simulink model "PPC_P2"  (R2019b)
settings: Solver=VariableStepAuto  StartTime=0.0  StopTime=50.0  RelTol=1e-3
undefined symbols (not defined in the file): sigbuilder_block
libraries: slctrlblks x2, simulink x1
settings Model: Creator=Kevin  LastModifiedBy=Kevin

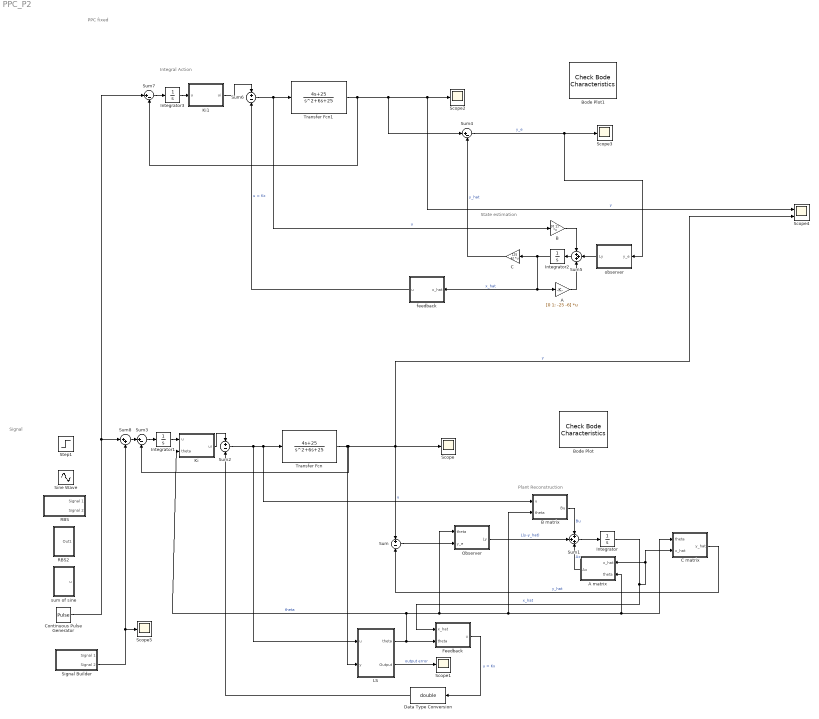
== system PPC_P2 ==
  note: PPC fixed
  note: Plant Reconstruction
  note: Signal
  note: Integral Action
  note: State estimation
  A : Gain  Gain=[0 1; -25 -6]  Multiplication=Matrix(K*u)
  A matrix : MATLAB Function  TreatAsAtomicUnit=on
  B : Gain  Gain=[0 1]'  Multiplication=Matrix(K*u)
  B matrix : MATLAB Function  TreatAsAtomicUnit=on
  Bode Plot : slctrlblks/Model Verification/Check Bode  Characteristics  InstantiateOnLoad=on  SaveOperatingPoints=off  LinearizationIOs={'/Sum2', 1, 'in', 'on', '';'/Transfer Fcn', 1, 'out', 'on', ''}  LinearizeAt=SnapshotTimes  SnapshotTimes=[0]  TriggerType=rising  SampleTime=auto  RateConversionMethod=zoh  PreWarpFreq=10  UseExactDelayModel=off  UseFullBlockNameLabels=off  UseBusSignalLabels=off  enabled=on  stopWhenAssertionFail=off  export=off  ViewDlgPos=[1921 -319 1920 967.333333333333]  OpenViewOnLoad=off  LaunchViewOnOpen=off  FrequencyUnits=rad/s  MagnitudeUnits=dB  PhaseUnits=deg  TimeUnits=seconds  EnableUpperBound=off  UpperBoundFrequencies=[]  UpperBoundMagnitudes=[]  EnableLowerBound=off  LowerBoundFrequencies=[]  LowerBoundMagnitudes=[]
      settings: SourceProductName=Simulink Control Design
  Bode Plot1 : slctrlblks/Model Verification/Check Bode  Characteristics  InstantiateOnLoad=on  SaveOperatingPoints=off  LinearizationIOs={'/Sum2', 1, 'in', 'off', '';'/Transfer Fcn', 1, 'out', 'on', ''}  LinearizeAt=SnapshotTimes  SnapshotTimes=[0]  TriggerType=rising  SampleTime=auto  RateConversionMethod=zoh  PreWarpFreq=10  UseExactDelayModel=off  UseFullBlockNameLabels=off  UseBusSignalLabels=off  enabled=on  stopWhenAssertionFail=off  export=off  ViewDlgPos=[1921 -319 1920 967.333333333333]  OpenViewOnLoad=off  LaunchViewOnOpen=off  FrequencyUnits=rad/s  MagnitudeUnits=dB  PhaseUnits=deg  TimeUnits=seconds  EnableUpperBound=off  UpperBoundFrequencies=[]  UpperBoundMagnitudes=[]  EnableLowerBound=off  LowerBoundFrequencies=[]  LowerBoundMagnitudes=[]
      settings: SourceProductName=Simulink Control Design
  C : Gain  Gain=[25 4]  Multiplication=Matrix(K*u)
  C matrix : MATLAB Function  TreatAsAtomicUnit=on
  Continuous Pulse Generator : DiscretePulseGenerator  PulseType=Time based  Period=1  PulseWidth=50
  Data Type Conversion : DataTypeConversion  OutDataTypeStr=double
  Feedback : MATLAB Function  TreatAsAtomicUnit=on
  Integrator{,1..3} (4 alike) : Integrator
  Ki : MATLAB Function  TreatAsAtomicUnit=on
  Ki1 : MATLAB Function  TreatAsAtomicUnit=on
  LS : Subsystem
  "Observer " : MATLAB Function  TreatAsAtomicUnit=on
  "RBS " : Subsystem  Tag=STV Subsys  LoadFcn=sigbuilder_block('load');  StartFcn=sigbuilder_block('start');  StopFcn=sigbuilder_block('stop');  ClipboardFcn=sigbuilder_block('clipboard');  mask(Sigbuilder block){tuvar=[0:10]}
      mask help: Simulink:masks:SigbuilderBlock_MD
      mask init:
      | if ~strcmp(get_param(bdroot(gcbh),'SimulationStatus'),'stopped') tuvar = sigbuilder_block('maskInit'); end
      settings: CopyFcn=sigbuilder_block('copy');  DeleteFcn=sigbuilder_block('delete');  ModelCloseFcn=sigbuilder_block('modelClose');  PreSaveFcn=sigbuilder_block('preSave');  PauseFcn=sigbuilder_block('pause');  ContinueFcn=sigbuilder_block('continue');  NameChangeFcn=sigbuilder_block('namechange');  OpenFcn=sigbuilder_block('open',[215 62.5 550.5 362.5 ]);  CloseFcn=sigbuilder_block('close');
      mask Display: plot(0, 0, 100, 100,[2, 2, 32, 32, 2], [68, 8, 8, 68, 68],[32, 2], [38, 38], [32, 19, 2],[53, 60, 44], [32, 17, 17, 2],[16, 16, 31, 31]);txt = getActiveGroup(gcbh);text(2, 100, txt,'verticalAlignment', 'top');
  RBS2 : Subsystem
  Scope{,1..3,5} (5 alike) : Scope
  Scope4 : Scope  NumInputPorts=2
  Signal Builder : Subsystem  Tag=STV Subsys  LoadFcn=sigbuilder_block('load',[242.5 79.5 550.5 362.5 ]);  StartFcn=sigbuilder_block('start');  StopFcn=sigbuilder_block('stop');  ClipboardFcn=sigbuilder_block('clipboard');  mask(Sigbuilder block){tuvar=[0:10]}
      mask help: Simulink:masks:SigbuilderBlock_MD
      mask init:
      | if ~strcmp(get_param(bdroot(gcbh),'SimulationStatus'),'stopped') tuvar = sigbuilder_block('maskInit'); end
      settings: CopyFcn=sigbuilder_block('copy');  DeleteFcn=sigbuilder_block('delete');  ModelCloseFcn=sigbuilder_block('modelClose');  PreSaveFcn=sigbuilder_block('preSave');  PauseFcn=sigbuilder_block('pause');  ContinueFcn=sigbuilder_block('continue');  NameChangeFcn=sigbuilder_block('namechange');  OpenFcn=sigbuilder_block('open',[216 79 550.5 362.5 ]);  CloseFcn=sigbuilder_block('close');
      mask Display: plot(0, 0, 100, 100,[2, 2, 32, 32, 2], [68, 8, 8, 68, 68],[32, 2], [38, 38], [32, 19, 2],[53, 60, 44], [32, 17, 17, 2],[16, 16, 31, 31]);txt = getActiveGroup(gcbh);text(2, 100, txt,'verticalAlignment', 'top');
  Sine Wave : Sin  Frequency=0.1  SampleTime=0
  Step1 : Step  SampleTime=0
  Sum : Sum  Inputs=+-
  Sum1 : Sum  Inputs=+++
  Sum2 : Sum  Inputs=+-
  Sum3 : Sum  Inputs=|+-
  Sum4 : Sum  Inputs=|+-
  Sum5 : Sum  Inputs=+++
  Sum6 : Sum  Inputs=+-
  Sum7 : Sum  Inputs=|+-
  Sum8 : Sum  Inputs=|++
  Transfer Fcn : TransferFcn  Numerator=[4 25]  Denominator=[1 ,6 ,25]
  Transfer Fcn1 : TransferFcn  Numerator=[4 25]  Denominator=[1 ,6 ,25]
  feedback : MATLAB Function  TreatAsAtomicUnit=on
  "observer " : MATLAB Function  TreatAsAtomicUnit=on
  sum of sine : Subsystem
  wires:
  "Observer "/1(Ly) -> Sum1/2  "L(y-y_hat)"
  LS/2(Output) -> Scope1/1  "output error"
  B matrix/1(Bu) -> Sum1/1  "Bu"
  Sum1/1 -> Integrator/1
  LS/1(theta) -> C matrix/1(theta), A matrix/2(theta), B matrix/2(theta), "Observer "/1(theta), Ki/2(theta), Feedback/2(theta)  "theta"
  A matrix/1(Ax) -> Sum1/3  "Ax"
  Integrator/1 -> C matrix/2(x_hat), A matrix/1(x_hat), Feedback/1(x_hat)  "x_hat"
  Sum2/1 -> LS/1("u "), B matrix/1(u), Transfer Fcn/1  "u"
  Sum/1 -> "Observer "/2(y_e)
  Transfer Fcn/1 -> Sum/1, Scope4/2, Scope/1, Sum3/2, LS/2(y)  "y"
  Feedback/1(u) -> Data Type Conversion/1  "u = Kx"
  C matrix/1(y_hat) -> Sum/2  "y_hat"
  Data Type Conversion/1 -> Sum2/2
  Sum3/1 -> Integrator1/1
  Integrator1/1 -> Ki/1(u)
  Ki/1(ui) -> Sum2/1
  feedback/1(u) -> Sum6/2  "u = Kx"
  Sum4/1 -> "observer "/1(y_e), Scope3/1  "y_e"
  Ki1/1(ui) -> Sum6/1
  Integrator3/1 -> Ki1/1(u)
  Transfer Fcn1/1 -> Sum4/1, Scope4/1, Scope2/1, Sum7/2  "y"
  A/1 -> Sum5/3
  Integrator2/1 -> C/1, feedback/1(x_hat), A/1  "x_hat"
  Sum5/1 -> Integrator2/1
  C/1 -> Sum4/2  "y_hat"
  "observer "/1(Ly) -> Sum5/2
  Sum7/1 -> Integrator3/1
  B/1 -> Sum5/1
  Continuous Pulse Generator/1 -> Sum8/1, Sum7/1
  Sum6/1 -> B/1, Transfer Fcn1/1  "u"
  Sum8/1 -> Sum3/1
  Signal Builder/2(Signal 2) -> Scope5/1, Sum8/2

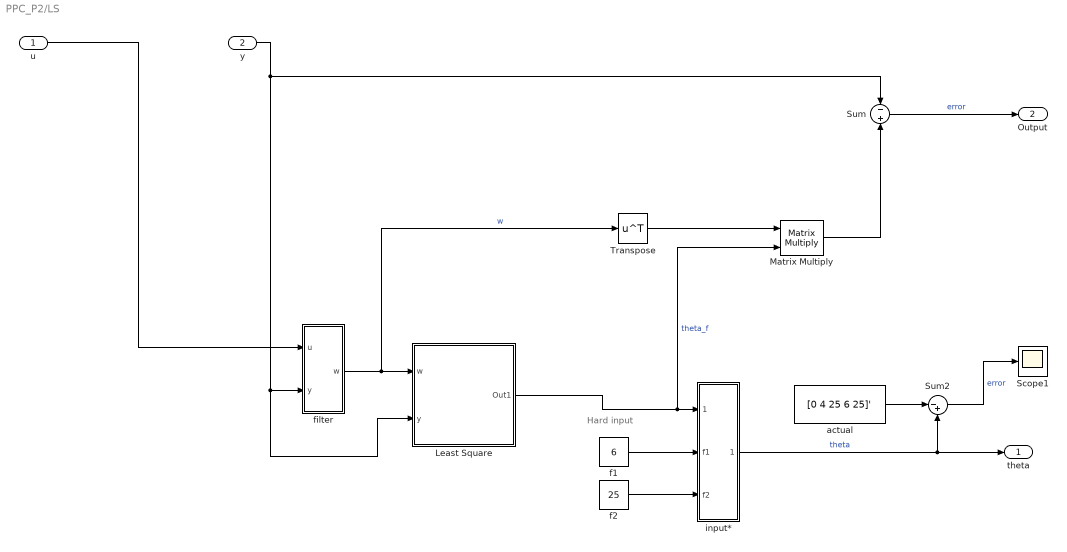
== system PPC_P2/LS ==
  note: Hard input
  "u " : Inport
  y : Inport  Port=2
  Least Square : Subsystem
  Matrix Multiply : Product  Multiplication=Matrix(*)
  Scope1 : Scope
  Sum : Sum  Inputs=-+
  Sum2 : Sum  Inputs=|-+
  Transpose : Math  Operator=transpose  SignedPower=off  SaturateOnIntegerOverflow=on
  actual : Constant  Value=[0 4 25 6 25]'
  f1 : Constant  Value=6
  f2 : Constant  Value=25
  "filter " : Subsystem
  input* : Subsystem
  theta : Outport
  Output : Outport  Port=2
  wires:
  y/1 -> Sum/1, Least Square/2(y), "filter "/2("y ")
  Sum2/1 -> Scope1/1  "error"
  f2/1 -> input*/3(f2)
  actual/1 -> Sum2/1
  "u "/1 -> "filter "/1("u ")
  f1/1 -> input*/2(f1)
  Least Square/1(Out1) -> Matrix Multiply/2, input*/1(theta_f)  "theta_f"
  input*/1(Out1) -> Sum2/2, theta/1  "theta"
  "filter "/1(w) -> Transpose/1, Least Square/1(w)  "w"
  Transpose/1 -> Matrix Multiply/1
  Matrix Multiply/1 -> Sum/2
  Sum/1 -> Output/1  "error"

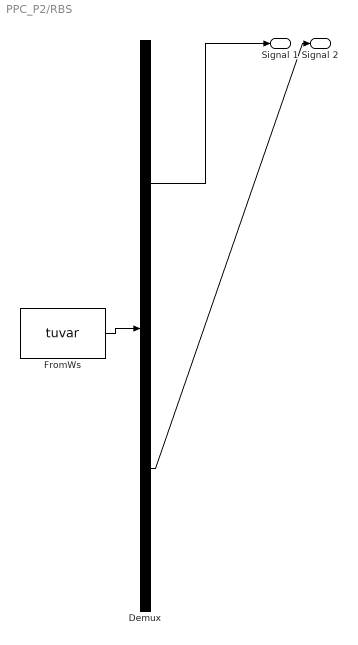
== system PPC_P2/RBS  ==
  Demux : Demux  Tag=STV Demux  Outputs=2
  FromWs : FromWorkspace  Tag=STV FromWs  VariableName=tuvar  SampleTime=0
      SigBuilderData=|
      | common.afterFinalStr = 'Extrapolate'
      | common.sampleTime = 0
      | dataSet.timeRange = [0 10]
      | dataSet.name = 'Group 1'
      | sbobj.Groups.Name = 'Group 1'
      | sbobj.Groups.Signals(1).Name = 'Signal 1'
      | sbobj.Groups.Signals(1).XData = [0 4 4 6 6 10]
      | sbobj.Groups.Signals(1).YData = [0 0 1 1 0 0]
      | sbobj.Groups.Signals(2).Name = 'Signal 2'
      | sbobj.Groups.Signals(2).XData = [0 0.2 0.2 0.3 0.3 0.5 0.5 0.7 0.7 1 1 1.1 1.1 1.3 1.3 1.4 1.4 1.5 1.5 1.7 1.7 2.1 2.1 2.2 2.2 2.7 2.7 2.8 2.8 2.9 2.9 3 3 3.1 3.1 3.5 3.5 3.7 3.7 3.8 3.8 3.9 3.9 4.2 4.2 4.4 4.4 4.7 4.7 5 5 5.1 5.1 5.3 5.3 5.6 5.6 5.7 5.7 5.8 5.8 5.9 5.9 6 6 6.1 6.1 6.2 6.2 6.7 6.7 7 7 7.1 7.1 7.2 7.2 7.3 7.3 7.4 7.4 7.5 7.5 7.8 7.8 7.9 7.9 8.1 8.1 8.5 8.5 8.6 8.6 8.8 8.8 8.9 8.9 9 9 9.2 9.2 9.5 9.5 9.6 9.6 9.7 9.7 10]
      | sbobj.Groups.Signals(2).YData = [1 1 0 0 1 1 0 0 1 1 0 0 1 1 0 0 1 1 0 0 1 1 0 0 1 1 0 0 1 1 0 0 1 1 0 0 1 1 0 0 1 1 0 0 1 1 0 0 1 1 0 0 1 1 0 0 1 1 0 0 1 1 0 0 1 1 0 0 1 1 0 0 1 1 0 0 1 1 0 0 1 1 0 0 1 1 0 0 1 1 0 0 1 1 0 0 1 1 0 0 1 1 0 0 1 1 0 0]
  Signal 1 : Outport  Tag=STV Outport
  Signal 2 : Outport  Tag=STV Outport  Port=2
  wires:
  Demux/1 -> Signal 1/1
  FromWs/1 -> Demux/1
  Demux/2 -> Signal 2/1

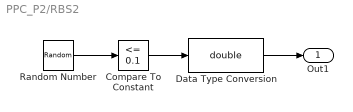
== system PPC_P2/RBS2 ==
  Compare To Constant : simulink/Logic and Bit Operations/Compare To Constant  relop=<=  const=0.1  OutDataTypeStr=boolean
  Data Type Conversion : DataTypeConversion  OutDataTypeStr=double
  Random Number : RandomNumber  Mean=1  SampleTime=10
  Out1 : Outport
  wires:
  Random Number/1 -> Compare To Constant/1
  Compare To Constant/1 -> Data Type Conversion/1
  Data Type Conversion/1 -> Out1/1

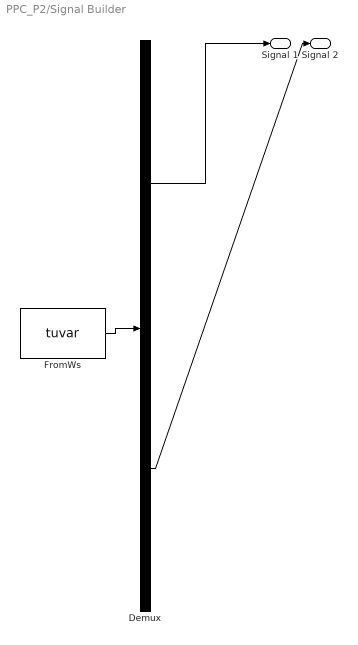
== system PPC_P2/Signal Builder ==
  Demux : Demux  Tag=STV Demux  Outputs=2
  FromWs : FromWorkspace  Tag=STV FromWs  VariableName=tuvar  SampleTime=0
      SigBuilderData=|
      | common.afterFinalStr = 'Extrapolate'
      | common.sampleTime = 0
      | dataSet.timeRange = [0 10]
      | dataSet.name = 'Group 1'
      | sbobj.Groups.Name = 'Group 1'
      | sbobj.Groups.Signals(1).Name = 'Signal 1'
      | sbobj.Groups.Signals(1).XData = [0 4 4 6 6 10]
      | sbobj.Groups.Signals(1).YData = [0 0 1 1 0 0]
      | sbobj.Groups.Signals(2).Name = 'Signal 2'
      | sbobj.Groups.Signals(2).XData = [0 0.25 0.5 0.75 1 1.25 1.5 1.75 2 2.25 2.5 2.75 3 3.25 3.5 3.75 4 4.25 4.5 4.75 5 5.25 5.5 5.75 6 6.25 6.5 6.75 7 7.25 7.5 7.75 8 8.25 8.5 8.75 9 9.25 9.5 9.75 10]
      | sbobj.Groups.Signals(2).YData = [0.0121419340162 -0.0764190690584 -0.164320775559 0.502978184919 0.351900863104 -0.0567183942106 0.0259717929394 0.453768030385 0.537981216054 0.330786163264 -0.0977542366685 -0.174844476245 0.225476170998 -0.259120295299 -0.321262673984 -0.106571039605 0.286763871566 0.0477844956174 0.0734825422898 0.33742490315 0.0703883754895 -0.341568743769 0.252628091547 0.142902550846 -0.0265169068696 -0.123910688666 -0.16337499212 -0.00720200578647 -0.240154097162 -0.153657109632 -0.446002612072 -0.155592567203 -0.207968715344 0.173295533063 0.436490088667 0.310645454952 0.314047045754 0.202863163156 0.16397838294 0.224996602257 -0.218951692736]
  Signal 1 : Outport  Tag=STV Outport
  Signal 2 : Outport  Tag=STV Outport  Port=2
  wires:
  Demux/1 -> Signal 1/1
  FromWs/1 -> Demux/1
  Demux/2 -> Signal 2/1

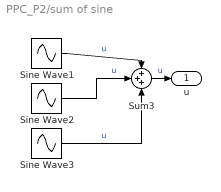
== system PPC_P2/sum of sine ==
  Sine Wave1 : Sin  Frequency=0.1  Phase=0.1  SampleTime=0
  Sine Wave2 : Sin  SampleTime=0
  Sine Wave3 : Sin  Frequency=2  SampleTime=0
  Sum3 : Sum  Inputs=+++
  u : Outport
  wires:
  Sine Wave3/1 -> Sum3/3  "u"
  Sine Wave1/1 -> Sum3/1  "u"
  Sum3/1 -> u/1  "u"
  Sine Wave2/1 -> Sum3/2  "u"

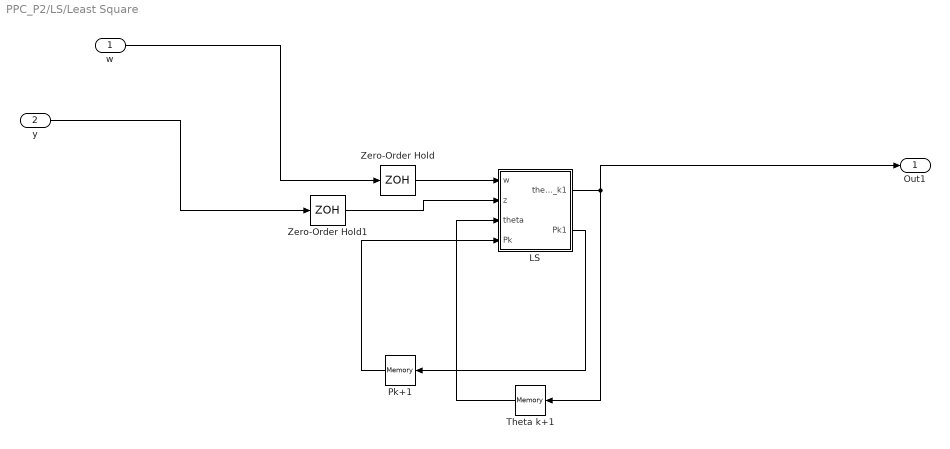
== system PPC_P2/LS/Least Square ==
  w : Inport
  y : Inport  Port=2
  LS : MATLAB Function  TreatAsAtomicUnit=on
  Pk+1 : Memory  InitialCondition=(10^5)*eye(5)  InheritSampleTime=on
  Theta k+1 : Memory  InitialCondition=[0 4.4 27.5 0.1 0.1]'  InheritSampleTime=on
  Zero-Order Hold : ZeroOrderHold  SampleTime=0.01
  Zero-Order Hold1 : ZeroOrderHold  SampleTime=0.01
  Out1 : Outport
  wires:
  Zero-Order Hold/1 -> LS/1(w)
  Pk+1/1 -> LS/4(Pk)
  Zero-Order Hold1/1 -> LS/2(z)
  LS/1(theta_k1) -> Out1/1, Theta k+1/1
  y/1 -> Zero-Order Hold1/1
  LS/2(Pk1) -> Pk+1/1
  Theta k+1/1 -> LS/3(theta)
  w/1 -> Zero-Order Hold/1

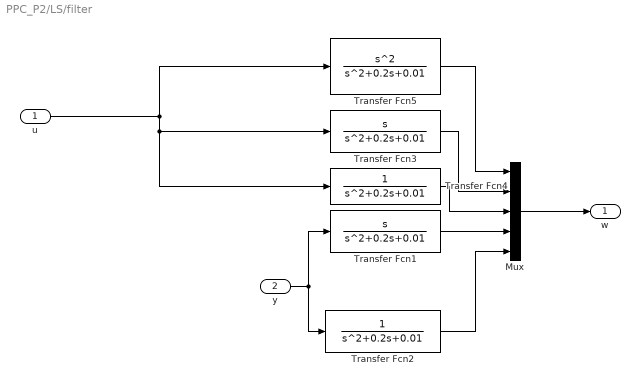
== system PPC_P2/LS/filter  ==
  "u " : Inport
  "y " : Inport  Port=2
  Mux : Mux  Inputs=5
  Transfer Fcn1 : TransferFcn  Numerator=[1 0]  Denominator=[1 0.2 0.01]
  Transfer Fcn2 : TransferFcn  Denominator=[1 0.2 0.01]
  Transfer Fcn3 : TransferFcn  Numerator=[1 0]  Denominator=[1 0.2 0.01]
  Transfer Fcn4 : TransferFcn  Denominator=[1 0.2 0.01]
  Transfer Fcn5 : TransferFcn  Numerator=[1 0 0]  Denominator=[1 0.2 0.01]
  w : Outport
  wires:
  Transfer Fcn1/1 -> Mux/4
  "u "/1 -> Transfer Fcn4/1, Transfer Fcn3/1, Transfer Fcn5/1
  Mux/1 -> w/1
  "y "/1 -> Transfer Fcn1/1, Transfer Fcn2/1
  Transfer Fcn2/1 -> Mux/5
  Transfer Fcn5/1 -> Mux/1
  Transfer Fcn3/1 -> Mux/2
  Transfer Fcn4/1 -> Mux/3

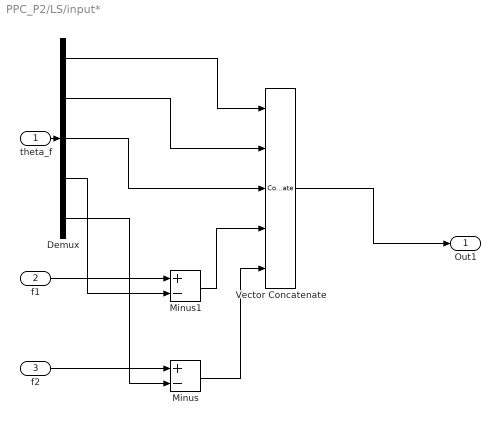
== system PPC_P2/LS/input* ==
  theta_f : Inport
  f1 : Inport  Port=2
  f2 : Inport  Port=3
  Demux : Demux  Outputs=5
  Minus : Sum  Inputs=+-
  Minus1 : Sum  Inputs=+-
  Vector Concatenate : Concatenate  NumInputs=5
  Out1 : Outport
  wires:
  Vector Concatenate/1 -> Out1/1
  Minus1/1 -> Vector Concatenate/4
  Minus/1 -> Vector Concatenate/5
  Demux/1 -> Vector Concatenate/1
  Demux/4 -> Minus1/2
  Demux/3 -> Vector Concatenate/3
  Demux/5 -> Minus/2
  f2/1 -> Minus/1
  Demux/2 -> Vector Concatenate/2
  f1/1 -> Minus1/1
  theta_f/1 -> Demux/1

== matlab function PPC_P2/LS/Least Square/LS ==
  data: w input; z input; theta input; Pk input; theta_k1 output; Pk1 output
function [ theta_k1,Pk1] = fcn(w, z, theta, Pk)
alpha = 1.4; %standard
gamma = 1/alpha;
%e = 10^-4;
%Q = e*eye(5);
%Pk = eye(5);

%initial values
%ro = 10^5;
%P1 = ro*eye(5);
%theta1 = [0 0 1 0.2 0.01]';
%Calculations

theta_k1 = theta - (gamma*Pk*w*(w'*theta-z))/ (1+gamma*w'*Pk*w);
Pk1 = (1/alpha)*Pk - ((gamma^2*Pk*w*w'*Pk)/(1+gamma*w'*Pk*w));

== matlab function PPC_P2/Ki ==
  data: u input; ui output; theta input
function ui = fcn(u , theta)
 coder.extrinsic("ss","place","matsplit",'ctrb');
% [b2, b1, b0, a1, a0] = matsplit(theta);
ui = 0;
A = [0 1; -theta(5) -theta(4)];
B = [0 1]';
C = [theta(3) theta(2)];
% D = 0;

o = [0 0]';
A1 = [A o;C 0];
B1 = [B;0];
p = [-30+4i -30-4i -10]; %let third pole be less affective
K1 = place(A1,B1,p);
Ki = [K1(3)];
ui = Ki*u;

== matlab function PPC_P2/Ki1 ==
  data: u input; ui output
function ui = fcn(u)
 coder.extrinsic("ss","place","matsplit",'ctrb');
% [b2, b1, b0, a1, a0] = matsplit(theta);
ui = 0;
A = [0 1; -25 -6];
B = [0 1]';
C = [25 4]; 

o = [0 0]';
A1 = [A o;C 0];
B1 = [B;0];
p = [-30+4i -30-4i -10]; %let third pole be less affective
K1 = place(A1,B1,p);
Ki = [K1(3)];
ui = Ki*u;

== matlab function PPC_P2/Feedback ==
  data: x_hat input; theta input; u output
function u = fcn(x_hat, theta)
 coder.extrinsic("ss","place","matsplit",'ctrb');
% [b2, b1, b0, a1, a0] = matsplit(theta);
u = 0;
A = [0 1; -theta(5) -theta(4)];
B = [0 1]';
C = [theta(3) theta(2)];
% D = 0;

%pole design
% %sys = ss(A,B,C,D);
% p = [-.1+0.7071i -.1-0.7071i];
% K = place(A,B,p);
% a0 = theta(5); a1 = theta(4); 
% p1 = -30; p2 = -30; 
% alpha = [-(p1+p2) p1*p2];
% P = ctrb(A,B);
% Pccf1 = [a1 1; 1 0];
% K = [alpha(2)-a0 alpha(1)-a1]*inv(P*Pccf1);

%servomechanism
o = [0 0]';
A1 = [A o;C 0];
B1 = [B;0];
p = [-30+4i -30-4i -10]; %let third pole be less affective
K1 = place(A1,B1,p);
K = [K1(1) K1(2)];

u = K*x_hat;

== matlab function PPC_P2/Observer  ==
  data: theta input; y_e input; Ly output
function Ly = fcn(theta, y_e)
 coder.extrinsic('ss','place','pole','matsplit','complex','real','imag','ctrb');
 Ly = [0 0];
% %place pole 10 times to the left from the actual plant
% %[b2, b1, b0, a1, a0] = matsplit(theta);
A = [0 1; -theta(5) -theta(4)];
B = [0 1]';
C = [theta(3) theta(2)];
%sys = ss(A,B,C,0);
%p = pole(sys);
%p_des = [complex(10*real(p(1)),imag(p(1))) complex(10*real(p(2)),imag(p(2)))];
% p1 = complex(10*real(p(1)),imag(p(1)));
% p2 = complex(10*real(p(2)),imag(p(2)));
% p_des = [-10+i -10-i];
% L = place(A,C,p_des);
% p1 = real(p(1))*10;
% p2 = real(p(2))*10;
a0 = theta(5);
a1 = theta(4);
P = ctrb(A,B);
Pccf1 = [a1 1; 1 0];
p1 = -300; p2 = -300; 
alpha = [-(p1+p2) p1*p2];

L = [alpha(2)-a0 alpha(1)-a1]*inv(P*Pccf1);
Ly = L*y_e;

== matlab function PPC_P2/feedback ==
  data: x_hat input; u output
function u = fcn(x_hat)
 coder.extrinsic("ss","place","matsplit",'ctrb');
% [b2, b1, b0, a1, a0] = matsplit(theta);
%[0 4 25 6 25]
% A = [0 1; -theta(5) -theta(4)];
% B = [0 1]';
% C = [theta(3) theta(2)];

K = [0 0];
u = 0;
A = [0 1; -25 -6];
B = [0 1]';
C = [25 4]; 

%servomechanism
o = [0 0]';
A1 = [A o;C 0];
B1 = [B;0];
%p = [-30+0.01i -30-0.01i -0.15]; %let third pole be less affective
p = [-30+4i -30-4i -10];
K1 = place(A1,B1,p);
K = [K1(1) K1(2)];
u = K*x_hat;

== matlab function PPC_P2/C matrix ==
  data: theta input; x_hat input; y_hat output
function y_hat = fcn(theta, x_hat)
%coder.extrinsic("matsplit");
%[b2, b1, b0, a1, a0] = matsplit(theta);
%C = [b0 b1];
C = [theta(3) theta(2)];
y_hat = C*x_hat;

== matlab function PPC_P2/A matrix ==
  data: x_hat input; Ax output; theta input
function Ax = fcn(x_hat, theta)
%coder.extrinsic("matsplit");
%[b2, b1, b0, a1, a0] = matsplit(theta);
A = [0 1; -theta(5) -theta(4)];

Ax = A*x_hat;

== matlab function PPC_P2/B matrix ==
  data: u input; Bu output; theta input
function Bu = fcn(u, theta)
%coder.extrinsic("matsplit");
%[b2, b1, b0, a1, a0] = matsplit(theta);
B = [0 1]';
Bu = B*u;

== matlab function PPC_P2/observer  ==
  data: y_e input; Ly output
function Ly  = fcn(y_e)
coder.extrinsic("ss","place","matsplit",'ctrb');
Ly = [0 0];
A = [0 1; -25 -6];
B = [0 1]';
C = [25 4]; 

%observer design
a0 = 25;
a1 = 6;
P = ctrb(A,B);
Pccf1 = [a1 1; 1 0];
p1 = -300; p2 = -300; 
alpha = [-(p1+p2) p1*p2];
L = [alpha(2)-a0 alpha(1)-a1]*inv(P*Pccf1);
Ly = L*y_e;
